simulink model "Model_6DOF_B3"  (R2020b)
settings: Solver=FixedStepAuto  StartTime=0.0  StopTime=120  FixedStep=0.05  RelTol=1e-3
values from neighbouring files (symbols this model uses):
  Ba_0 = [0 0 0 0 0 0]    [ctrl_mode_param.m]
  Bb = 4418825.3321    [load_data.m]
  Bv_0 = [tgt_speed 0 0 0 0 0]    [ctrl_mode_param.m]
  Bx_0 = [0 0 tgt_depth 0 0 0]    [ctrl_mode_param.m]
  Ixx = 5.23e7    (= 52300000)    [load_data.m]
  Ixy = 0    [load_data.m]
  Ixz = 0    [load_data.m]
  Iyy = 1.375e9    (= 1375000000)    [load_data.m]
  Iyz = 0    [load_data.m]
  Izz = 1.367e9    (= 1367000000)    [load_data.m]
  Mb = 4418825.3321    [load_data.m]
  Xb = 0    [load_data.m]
  Xg = 0    [load_data.m]
  Yb = 0    [load_data.m]
  Yg = 0    [load_data.m]
  Zb = 0.4406    [load_data.m]
  Zg = 0    [load_data.m]
undefined symbols (not defined in the file or in its folder): dA_BP1, dA_BP2, dA_Hull, dA_PH, dA_Sail, dA_SProot, dA_X1a, dA_X1b, dA_X2a, dA_X2b, dA_X3a, dA_X3b, dA_X4a, dA_X4b, its, n_BP1, n_BP2, n_Hull, n_PH, n_Sail, n_SProot, n_X1a, n_X1b, n_X2a, n_X2b, n_X3a, n_X3b, n_X4a, n_X4b, nt_BP1, nt_BP2, nt_Hull, nt_PH, nt_Sail, nt_SProot, nt_X1a, nt_X1b, nt_X2a, nt_X2b, nt_X3a, nt_X3b, nt_X4a, nt_X4b, Usp, vt1_BP1, vt1_BP2, vt1_Hull, vt1_PH, vt1_Sail, vt1_SProot, vt1_X1a, vt1_X1b, vt1_X2a, vt1_X2b, vt1_X3a, vt1_X3b, vt1_X4a, vt1_X4b, vt2_BP1, vt2_BP2 ... (+27)
libraries: simulink x5
(part 10 of 15)

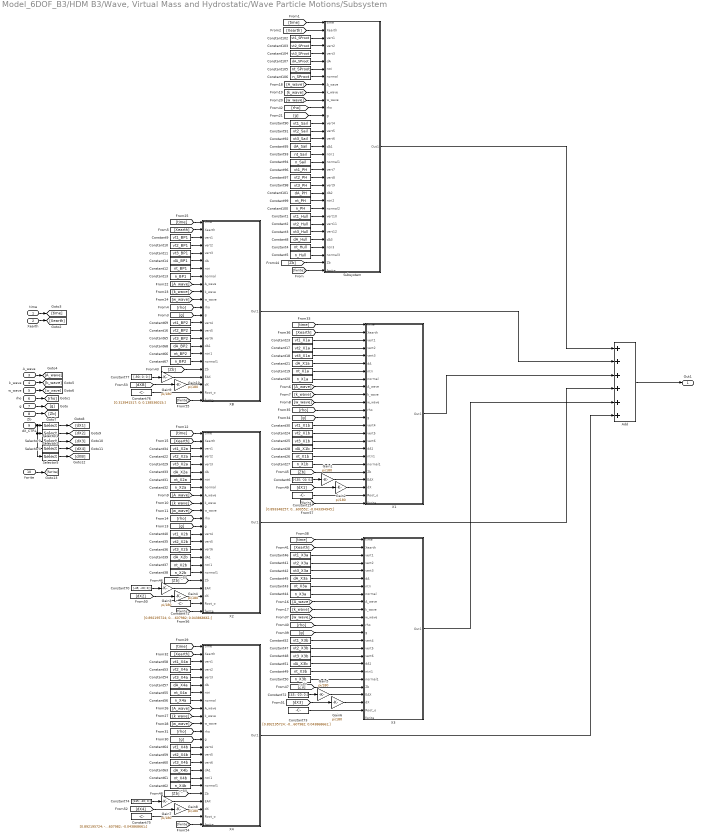
== system Model_6DOF_B3/HDM B3/Wave, Virtual Mass and Hydrostatic/Wave Particle Motions/Subsystem ==
  note: n_BP
  note: n_BP
  note: n_BP
  time : Inport
  Xearth : Inport  Port=2
  A_wave : Inport  Port=3
  k_wave : Inport  Port=4
  w_wave : Inport  Port=5
  rho : Inport  Port=6
  g : Inport  Port=7
  Zb : Inport  Port=8
  dX_CTRL : Inport  Port=9
  fwrite : Inport  Port=10
  Add : Sum  Inputs=6
  Constant1 : Constant  Value=vt1_Hull
  Constant10 : Constant  Value=vt2_BP1
  Constant100 : Constant  Value=n_PH
  Constant101 : Constant  Value=dA_PH
  Constant102 : Constant  Value=vt1_SProot
  Constant103 : Constant  Value=vt2_SProot
  Constant104 : Constant  Value=vt3_SProot
  Constant105 : Constant  Value=nt_SProot
  Constant106 : Constant  Value=n_SProot
  Constant107 : Constant  Value=dA_SProot
  Constant11 : Constant  Value=vt3_BP1
  Constant12 : Constant  Value=nt_BP1
  Constant13 : Constant  Value=n_BP1
  Constant14 : Constant  Value=dA_BP1
  Constant15 : Constant  Value=|
      | [0.893348257;
      | 0.043600552;
      | -0.043394945;]
  Constant16 : Constant  Value=vt2_BP2
  Constant17 : Constant  Value=vt2_X1a
  Constant18 : Constant  Value=vt3_X1a
  Constant19 : Constant  Value=nt_X1a
  Constant2 : Constant  Value=vt2_Hull
  Constant20 : Constant  Value=n_X1a
  Constant21 : Constant  Value=dA_X1a
  Constant22 : Constant  Value=vt2_X2a
  Constant23 : Constant  Value=vt1_X1a
  Constant24 : Constant  Value=vt2_X1b
  Constant25 : Constant  Value=vt3_X1b
  Constant26 : Constant  Value=nt_X1b
  Constant27 : Constant  Value=n_X1b
  Constant28 : Constant  Value=dA_X1b
  Constant29 : Constant  Value=vt3_X2a
  Constant3 : Constant  Value=vt3_Hull
  Constant30 : Constant  Value=vt1_X1b
  Constant31 : Constant  Value=nt_X2a
  Constant32 : Constant  Value=n_X2a
  Constant33 : Constant  Value=dA_X2a
  Constant34 : Constant  Value=vt1_X2a
  Constant35 : Constant  Value=vt2_X2b
  Constant36 : Constant  Value=vt3_X2b
  Constant37 : Constant  Value=nt_X2b
  Constant38 : Constant  Value=n_X2b
  Constant39 : Constant  Value=dA_X2b
  Constant4 : Constant  Value=nt_Hull
  Constant40 : Constant  Value=vt1_X2b
  Constant41 : Constant  Value=vt2_X3a
  Constant42 : Constant  Value=vt3_X3a
  Constant43 : Constant  Value=nt_X3a
  Constant44 : Constant  Value=n_X3a
  Constant45 : Constant  Value=dA_X3a
  Constant46 : Constant  Value=vt1_X3a
  Constant47 : Constant  Value=vt2_X3b
  Constant48 : Constant  Value=vt3_X3b
  Constant49 : Constant  Value=nt_X3b
  Constant5 : Constant  Value=n_Hull
  Constant50 : Constant  Value=n_X3b
  Constant51 : Constant  Value=dA_X3b
  Constant52 : Constant  Value=vt1_X3b
  Constant53 : Constant  Value=vt2_X4a
  Constant54 : Constant  Value=vt3_X4a
  Constant55 : Constant  Value=nt_X4a
  Constant56 : Constant  Value=n_X4a
  Constant57 : Constant  Value=dA_X4a
  Constant58 : Constant  Value=vt1_X4a
  Constant59 : Constant  Value=vt2_X4b
  Constant6 : Constant  Value=[-135; -20; 0;]
  Constant60 : Constant  Value=vt3_X4b
  Constant61 : Constant  Value=nt_X4b
  Constant62 : Constant  Value=n_X4b
  Constant63 : Constant  Value=dA_X4b
  Constant64 : Constant  Value=vt1_X4b
  Constant65 : Constant  Value=vt3_BP2
  Constant66 : Constant  Value=nt_BP2
  Constant67 : Constant  Value=n_BP2
  Constant68 : Constant  Value=dA_BP2
  Constant69 : Constant  Value=vt1_BP2
  Constant70 : Constant  Value=[-45; -20; 0;]
  Constant71 : Constant  Value=|
      | [0.892195724;
      | 0.043607982;
      | 0.043868661;]
  Constant72 : Constant  Value=[45; -20; 0;]
  Constant73 : Constant  Value=|
      | [0.892195724;
      | -0.043607982;
      | 0.043868661;]
  Constant74 : Constant  Value=[135; -20; 0;]
  Constant75 : Constant  Value=|
      | [0.892195724;
      | -0.043607982;
      | -0.043868661;]
  Constant76 : Constant  Value=|
      | [0.313941517;
      | 0;
      | 0.138536015;]
  Constant77 : Constant  Value=[-90; 0; 0;]
  Constant8 : Constant  Value=dA_Hull
  Constant9 : Constant  Value=vt1_BP1
  Constant90 : Constant  Value=vt1_Sail
  Constant91 : Constant  Value=vt2_Sail
  Constant92 : Constant  Value=vt3_Sail
  Constant93 : Constant  Value=nt_Sail
  Constant94 : Constant  Value=n_Sail
  Constant95 : Constant  Value=dA_Sail
  Constant96 : Constant  Value=vt1_PH
  Constant97 : Constant  Value=vt2_PH
  Constant98 : Constant  Value=vt3_PH
  Constant99 : Constant  Value=nt_PH
  Gain{1..10} (10 alike) : Gain  Gain=pi/180
  Selector1 : Selector  InputPortWidth=5  IndexOptions=Index vector (dialog)  Indices=1  OutputSizes=1
  Selector2 : Selector  InputPortWidth=5  IndexOptions=Index vector (dialog)  Indices=2  OutputSizes=1
  Selector3 : Selector  InputPortWidth=5  IndexOptions=Index vector (dialog)  Indices=3  OutputSizes=1
  Selector4 : Selector  InputPortWidth=5  IndexOptions=Index vector (dialog)  Indices=4  OutputSizes=1
  Selector5 : Selector  InputPortWidth=5  IndexOptions=Index vector (dialog)  Indices=5  OutputSizes=1
  Subsystem : Subsystem
  X1 : Subsystem
  X2 : Subsystem
  X3 : Subsystem
  X4 : Subsystem
  XB : Subsystem
  Out1 : Outport
  wires:
  time/1 -> [time]
  Xearth/1 -> [Xearth]
  A_wave/1 -> [A_wave]
  k_wave/1 -> [k_wave]
  w_wave/1 -> [w_wave]
  rho/1 -> [rho]
  g/1 -> [g]
  Constant94/1 -> Subsystem/19(normal1)
  Constant61/1 -> X4/18(ntri1)
  Constant57/1 -> X4/6(dA)
  [Zb] -> X4/20(Zb)
  [Zb] -> X3/20(Zb)
  Constant101/1 -> Subsystem/23(dA2)
  Constant16/1 -> XB/15(vert5)
  [Zb] -> X1/20(Zb)
  [Zb] -> X2/20(Zb)
  Constant98/1 -> Subsystem/22(vert9)
  Constant99/1 -> Subsystem/24(ntri2)
  Constant37/1 -> X2/18(ntri1)
  [Zb] -> XB/20(Zb)
  [time] -> X3/1(time)
  [Xearth] -> X1/2(Xearth)
  [w_wave] -> Subsystem/11(w_wave)
  Constant93/1 -> Subsystem/18(ntri1)
  [g] -> X2/13(g)
  Constant28/1 -> X1/17(dA1)
  [w_wave] -> X3/11(w_wave)
  Constant8/1 -> Subsystem/29(dA3)
  Constant95/1 -> Subsystem/17(dA1)
  [A_wave] -> X4/9(A_wave)
  Constant33/1 -> X2/6(dA)
  [rho] -> X4/12(rho)
  [time] -> Subsystem/1(time)
  Constant48/1 -> X3/16(vert6)
  [rho] -> Subsystem/12(rho)
  Constant60/1 -> X4/16(vert6)
  [k_wave] -> Subsystem/10(k_wave)
  Constant19/1 -> X1/7(ntri)
  [g] -> Subsystem/13(g)
  Constant102/1 -> Subsystem/3(vert1)
  Constant106/1 -> Subsystem/8(normal)
  [Xearth] -> Subsystem/2(Xearth)
  Constant107/1 -> Subsystem/6(dA)
  Constant105/1 -> Subsystem/7(ntri)
  [g] -> X4/13(g)
  Constant11/1 -> XB/5(vert3)
  Constant34/1 -> X2/3(vert1)
  Constant63/1 -> X4/17(dA1)
  [A_wave] -> X1/9(A_wave)
  Constant41/1 -> X3/4(vert2)
  [k_wave] -> X2/10(k_wave)
  Constant22/1 -> X2/4(vert2)
  Constant49/1 -> X3/18(ntri1)
  [Xearth] -> XB/2(Xearth)
  [rho] -> X2/12(rho)
  Constant27/1 -> X1/19(normal1)
  [rho] -> X3/12(rho)
  Constant55/1 -> X4/7(ntri)
  Constant45/1 -> X3/6(dA)
  Constant40/1 -> X2/14(vert4)
  Constant18/1 -> X1/5(vert3)
  [g] -> X1/13(g)
  Constant35/1 -> X2/15(vert5)
  Constant39/1 -> X2/17(dA1)
  Constant32/1 -> X2/8(normal)
  Constant47/1 -> X3/15(vert5)
  [w_wave] -> X4/11(w_wave)
  Constant44/1 -> X3/8(normal)
  [k_wave] -> X1/10(k_wave)
  Constant53/1 -> X4/4(vert2)
  [w_wave] -> XB/11(w_wave)
  [Xearth] -> X2/2(Xearth)
  [time] -> XB/1(time)
  [rho] -> XB/12(rho)
  Constant4/1 -> Subsystem/30(ntri3)
  Constant59/1 -> X4/15(vert5)
  Constant51/1 -> X3/17(dA1)
  Constant52/1 -> X3/14(vert4)
  Constant14/1 -> XB/6(dA)
  [Xearth] -> X3/2(Xearth)
  Constant25/1 -> X1/16(vert6)
  Constant67/1 -> XB/19(normal1)
  [Zb] -> Subsystem/32(Zb)
  Constant65/1 -> XB/16(vert6)
  Constant104/1 -> Subsystem/5(vert3)
  Constant13/1 -> XB/8(normal)
  Constant69/1 -> XB/14(vert4)
  Constant43/1 -> X3/7(ntri)
  [k_wave] -> X3/10(k_wave)
  [A_wave] -> X2/9(A_wave)
  Constant17/1 -> X1/4(vert2)
  [k_wave] -> XB/10(k_wave)
  Constant68/1 -> XB/17(dA1)
  Constant46/1 -> X3/3(vert1)
  Constant23/1 -> X1/3(vert1)
  Constant9/1 -> XB/3(vert1)
  Constant62/1 -> X4/19(normal1)
  [A_wave] -> XB/9(A_wave)
  Constant26/1 -> X1/18(ntri1)
  Constant56/1 -> X4/8(normal)
  Constant24/1 -> X1/15(vert5)
  Constant12/1 -> XB/7(ntri)
  Constant20/1 -> X1/8(normal)
  [g] -> X3/13(g)
  [w_wave] -> X1/11(w_wave)
  Constant100/1 -> Subsystem/25(normal2)
  Constant92/1 -> Subsystem/16(vert6)
  Constant30/1 -> X1/14(vert4)
  [time] -> X2/1(time)
  [rho] -> X1/12(rho)
  Constant91/1 -> Subsystem/15(vert5)
  [time] -> X1/1(time)
  Constant1/1 -> Subsystem/26(vert10)
  Constant31/1 -> X2/7(ntri)
  [w_wave] -> X2/11(w_wave)
  Constant21/1 -> X1/6(dA)
  Constant90/1 -> Subsystem/14(vert4)
  Constant96/1 -> Subsystem/20(vert7)
  Constant36/1 -> X2/16(vert6)
  Constant29/1 -> X2/5(vert3)
  [Xearth] -> X4/2(Xearth)
  Constant64/1 -> X4/14(vert4)
  Constant97/1 -> Subsystem/21(vert8)
  Constant2/1 -> Subsystem/27(vert11)
  Constant66/1 -> XB/18(ntri1)
  Constant54/1 -> X4/5(vert3)
  Constant38/1 -> X2/19(normal1)
  [k_wave] -> X4/10(k_wave)
  [time] -> X4/1(time)
  Constant10/1 -> XB/4(vert2)
  Constant50/1 -> X3/19(normal1)
  [A_wave] -> Subsystem/9(A_wave)
  Add/1 -> Out1/1
  Constant103/1 -> Subsystem/4(vert2)
  Constant3/1 -> Subsystem/28(vert12)
  [g] -> XB/13(g)
  Constant42/1 -> X3/5(vert3)
  Constant58/1 -> X4/3(vert1)
  Constant5/1 -> Subsystem/31(normal3)
  [A_wave] -> X3/9(A_wave)
  Zb/1 -> [Zb]
  Constant6/1 -> Gain1/1
  Gain1/1 -> X1/21(EAX)
  dX_CTRL/1 -> Selector2/1, Selector3/1, Selector5/1, Selector4/1, Selector1/1
  Selector1/1 -> [dX1]
  Selector2/1 -> [dX2]
  Selector3/1 -> [dX3]
  Selector4/1 -> [dX4]
  Selector5/1 -> [dXB]
  [dX1] -> Gain2/1
  Gain2/1 -> X1/22(dX)
  Constant15/1 -> X1/23(Root_o)
  Constant70/1 -> Gain3/1
  Gain3/1 -> X2/21(EAX)
  [dX2] -> Gain4/1
  Gain4/1 -> X2/22(dX)
  Constant71/1 -> X2/23(Root_o)
  Gain5/1 -> X3/21(EAX)
  [dX3] -> Gain6/1
  Constant72/1 -> Gain5/1
  Gain6/1 -> X3/22(dX)
  Constant73/1 -> X3/23(Root_o)
  Constant75/1 -> X4/23(Root_o)
  Gain7/1 -> X4/21(EAX)
  Constant74/1 -> Gain7/1
  [dX4] -> Gain8/1
  Gain8/1 -> X4/22(dX)
  Constant77/1 -> Gain9/1
  Gain9/1 -> XB/21(EAX)
  [dXB] -> Gain10/1
  Constant76/1 -> XB/23(Root_o)
  Gain10/1 -> XB/22(dX)
  [fwrite] -> Subsystem/33(fwrite)
  fwrite/1 -> [fwrite]
  [fwrite] -> X4/24(fwrite)
  [fwrite] -> XB/24(fwrite)
  [fwrite] -> X2/24(fwrite)
  [fwrite] -> X1/24(fwrite)
  X4/1(Out1) -> Add/6
  X3/1(Out1) -> Add/5
  X2/1(Out1) -> Add/4
  X1/1(Out1) -> Add/3
  XB/1(Out1) -> Add/2
  Subsystem/1(Out1) -> Add/1

== system Model_6DOF_B3/HDM B1/Wave, Virtual Mass and Hydrostatic/Wave Particle Motions/Subsystem/Sail Planes ==
  time : Inport
  Xearth : Inport  Port=2
  vert1 : Inport  Port=3
  vert2 : Inport  Port=4
  vert3 : Inport  Port=5
  dA : Inport  Port=6
  ntri : Inport  Port=7
  normal : Inport  Port=8
  A_wave : Inport  Port=9
  k_wave : Inport  Port=10
  w_wave : Inport  Port=11
  rho : Inport  Port=12
  g : Inport  Port=13
  vert4 : Inport  Port=14
  vert5 : Inport  Port=15
  vert6 : Inport  Port=16
  dA1 : Inport  Port=17
  ntri1 : Inport  Port=18
  normal1 : Inport  Port=19
  Zb : Inport  Port=20
  Add1 : Sum
  MATLAB Function1 : MATLAB Function  TreatAsAtomicUnit=on
  MATLAB Function2 : MATLAB Function  TreatAsAtomicUnit=on
  Mux1 : Mux  Inputs=6
  Mux2 : Mux  Inputs=6
  Out1 : Outport
  wires:
  Zb/1 -> MATLAB Function2/14(Zb), MATLAB Function1/14(Zb)
  vert6/1 -> MATLAB Function1/5(vert3)
  normal1/1 -> MATLAB Function1/8(normal)
  ntri1/1 -> MATLAB Function1/7(ntri)
  dA1/1 -> MATLAB Function1/6(dA)
  vert5/1 -> MATLAB Function1/4(vert2)
  vert2/1 -> MATLAB Function2/4(vert2)
  ntri/1 -> MATLAB Function2/7(ntri)
  normal/1 -> MATLAB Function2/8(normal)
  time/1 -> MATLAB Function2/1(time), MATLAB Function1/1(time)
  vert1/1 -> MATLAB Function2/3(vert1)
  Mux1/1 -> Add1/2
  vert3/1 -> MATLAB Function2/5(vert3)
  MATLAB Function1/6(Mz_total) -> Mux1/6
  Mux2/1 -> Add1/1
  MATLAB Function2/2(Fy_total) -> Mux2/2
  MATLAB Function2/6(Mz_total) -> Mux2/6
  g/1 -> MATLAB Function2/13(g), MATLAB Function1/13(g)
  k_wave/1 -> MATLAB Function1/10(k_wave), MATLAB Function2/10(k_wave)
  dA/1 -> MATLAB Function2/6(dA)
  vert4/1 -> MATLAB Function1/3(vert1)
  MATLAB Function2/5(My_total) -> Mux2/5
  MATLAB Function1/3(Fz_total) -> Mux1/3
  Add1/1 -> Out1/1
  MATLAB Function1/1(Fx_total) -> Mux1/1
  MATLAB Function2/1(Fx_total) -> Mux2/1
  MATLAB Function1/4(Mx_total) -> Mux1/4
  A_wave/1 -> MATLAB Function1/9(A_wave), MATLAB Function2/9(A_wave)
  rho/1 -> MATLAB Function2/12(rho), MATLAB Function1/12(rho)
  Xearth/1 -> MATLAB Function2/2(Xearth), MATLAB Function1/2(Xearth)
  MATLAB Function1/5(My_total) -> Mux1/5
  MATLAB Function1/2(Fy_total) -> Mux1/2
  w_wave/1 -> MATLAB Function2/11(w_wave), MATLAB Function1/11(w_wave)
  MATLAB Function2/4(Mx_total) -> Mux2/4
  MATLAB Function2/3(Fz_total) -> Mux2/3

== system Model_6DOF_B3/HDM B1/Wave, Virtual Mass and Hydrostatic/Wave Particle Motions/Subsystem/Subsystem ==
  time : Inport
  Xearth : Inport  Port=2
  vert1 : Inport  Port=3
  vert2 : Inport  Port=4
  vert3 : Inport  Port=5
  dA : Inport  Port=6
  ntri : Inport  Port=7
  normal : Inport  Port=8
  A_wave : Inport  Port=9
  k_wave : Inport  Port=10
  w_wave : Inport  Port=11
  rho : Inport  Port=12
  g : Inport  Port=13
  vert4 : Inport  Port=14
  vert5 : Inport  Port=15
  vert6 : Inport  Port=16
  dA1 : Inport  Port=17
  ntri1 : Inport  Port=18
  normal1 : Inport  Port=19
  vert7 : Inport  Port=20
  vert8 : Inport  Port=21
  vert9 : Inport  Port=22
  dA2 : Inport  Port=23
  ntri2 : Inport  Port=24
  normal2 : Inport  Port=25
  vert10 : Inport  Port=26
  vert11 : Inport  Port=27
  vert12 : Inport  Port=28
  dA3 : Inport  Port=29
  ntri3 : Inport  Port=30
  normal3 : Inport  Port=31
  Zb : Inport  Port=32
  Add1 : Sum  Inputs=4
  Constant : Constant
  Gain6 : Gain
  MATLAB Function1 : MATLAB Function  TreatAsAtomicUnit=on
  MATLAB Function2 : MATLAB Function  TreatAsAtomicUnit=on
  MATLAB Function3 : MATLAB Function  TreatAsAtomicUnit=on
  MATLAB Function4 : MATLAB Function  TreatAsAtomicUnit=on
  Mux{,1..3} (4 alike) : Mux  Inputs=6
  Out1 : Outport
  wires:
  Constant/1 -> MATLAB Function1/15(isample)
  Zb/1 -> MATLAB Function2/14(Zb), MATLAB Function1/14(Zb), MATLAB Function3/14(Zb), MATLAB Function4/14(Zb)
  vert8/1 -> MATLAB Function3/4(vert2)
  vert1/1 -> MATLAB Function2/3(vert1)
  vert10/1 -> MATLAB Function4/3(vert1)
  dA1/1 -> MATLAB Function1/6(dA)
  normal2/1 -> MATLAB Function3/8(normal)
  vert3/1 -> MATLAB Function2/5(vert3)
  vert6/1 -> MATLAB Function1/5(vert3)
  Add1/1 -> Out1/1
  vert2/1 -> MATLAB Function2/4(vert2)
  dA3/1 -> MATLAB Function4/6(dA)
  ntri3/1 -> MATLAB Function4/7(ntri)
  ntri2/1 -> MATLAB Function3/7(ntri)
  vert11/1 -> MATLAB Function4/4(vert2)
  MATLAB Function2/6(Mz_total) -> Mux3/6
  dA/1 -> MATLAB Function2/6(dA)
  Mux3/1 -> Gain6/1
  normal/1 -> MATLAB Function2/8(normal)
  MATLAB Function1/1(Fx_total) -> Mux1/1
  vert9/1 -> MATLAB Function3/5(vert3)
  Mux/1 -> Add1/4
  vert4/1 -> MATLAB Function1/3(vert1)
  MATLAB Function1/4(Mx_total) -> Mux1/4
  normal3/1 -> MATLAB Function4/8(normal)
  MATLAB Function3/5(My_total) -> Mux2/5
  vert12/1 -> MATLAB Function4/5(vert3)
  MATLAB Function2/1(Fx_total) -> Mux3/1
  MATLAB Function4/4(Mx_total) -> Mux/4
  dA2/1 -> MATLAB Function3/6(dA)
  MATLAB Function3/6(Mz_total) -> Mux2/6
  g/1 -> MATLAB Function2/13(g), MATLAB Function1/13(g), MATLAB Function3/13(g), MATLAB Function4/13(g)
  MATLAB Function3/3(Fz_total) -> Mux2/3
  ntri/1 -> MATLAB Function2/7(ntri)
  MATLAB Function3/2(Fy_total) -> Mux2/2
  MATLAB Function4/2(Fy_total) -> Mux/2
  Mux2/1 -> Add1/3
  MATLAB Function4/6(Mz_total) -> Mux/6
  MATLAB Function2/2(Fy_total) -> Mux3/2
  w_wave/1 -> MATLAB Function2/11(w_wave), MATLAB Function1/11(w_wave), MATLAB Function3/11(w_wave), MATLAB Function4/11(w_wave)
  MATLAB Function3/4(Mx_total) -> Mux2/4
  k_wave/1 -> MATLAB Function2/10(k_wave), MATLAB Function1/10(k_wave), MATLAB Function3/10(k_wave), MATLAB Function4/10(k_wave)
  MATLAB Function4/1(Fx_total) -> Mux/1
  MATLAB Function1/2(Fy_total) -> Mux1/2
  MATLAB Function2/3(Fz_total) -> Mux3/3
  MATLAB Function3/1(Fx_total) -> Mux2/1
  A_wave/1 -> MATLAB Function2/9(A_wave), MATLAB Function1/9(A_wave), MATLAB Function3/9(A_wave), MATLAB Function4/9(A_wave)
  MATLAB Function4/3(Fz_total) -> Mux/3
  normal1/1 -> MATLAB Function1/8(normal)
  Gain6/1 -> Add1/1
  MATLAB Function2/4(Mx_total) -> Mux3/4
  vert7/1 -> MATLAB Function3/3(vert1)
  MATLAB Function1/3(Fz_total) -> Mux1/3
  Mux1/1 -> Add1/2
  Xearth/1 -> MATLAB Function2/2(Xearth), MATLAB Function1/2(Xearth), MATLAB Function3/2(Xearth), MATLAB Function4/2(Xearth)
  MATLAB Function1/6(Mz_total) -> Mux1/6
  time/1 -> MATLAB Function2/1(time), MATLAB Function1/1(time), MATLAB Function3/1(time), MATLAB Function4/1(time)
  MATLAB Function2/5(My_total) -> Mux3/5
  MATLAB Function4/5(My_total) -> Mux/5
  vert5/1 -> MATLAB Function1/4(vert2)
  rho/1 -> MATLAB Function2/12(rho), MATLAB Function1/12(rho), MATLAB Function3/12(rho), MATLAB Function4/12(rho)
  MATLAB Function1/5(My_total) -> Mux1/5
  ntri1/1 -> MATLAB Function1/7(ntri)

== system Model_6DOF_B3/HDM B1/Wave, Virtual Mass and Hydrostatic/Wave Particle Motions/Subsystem/X1 ==
  time : Inport
  Xearth : Inport  Port=2
  vert1 : Inport  Port=3
  vert2 : Inport  Port=4
  vert3 : Inport  Port=5
  dA : Inport  Port=6
  ntri : Inport  Port=7
  normal : Inport  Port=8
  A_wave : Inport  Port=9
  k_wave : Inport  Port=10
  w_wave : Inport  Port=11
  rho : Inport  Port=12
  g : Inport  Port=13
  vert4 : Inport  Port=14
  vert5 : Inport  Port=15
  vert6 : Inport  Port=16
  dA1 : Inport  Port=17
  ntri1 : Inport  Port=18
  normal1 : Inport  Port=19
  Zb : Inport  Port=20
  Add1 : Sum
  MATLAB Function1 : MATLAB Function  TreatAsAtomicUnit=on
  MATLAB Function2 : MATLAB Function  TreatAsAtomicUnit=on
  Mux1 : Mux  Inputs=6
  Mux2 : Mux  Inputs=6
  Out1 : Outport
  wires:
  MATLAB Function1/3(Fz_total) -> Mux2/3
  MATLAB Function1/4(Mx_total) -> Mux2/4
  w_wave/1 -> MATLAB Function1/11(w_wave), MATLAB Function2/11(w_wave)
  MATLAB Function2/2(Fy_total) -> Mux1/2
  MATLAB Function2/5(My_total) -> Mux1/5
  Xearth/1 -> MATLAB Function2/2(Xearth), MATLAB Function1/2(Xearth)
  rho/1 -> MATLAB Function2/12(rho), MATLAB Function1/12(rho)
  A_wave/1 -> MATLAB Function1/9(A_wave), MATLAB Function2/9(A_wave)
  MATLAB Function2/4(Mx_total) -> Mux1/4
  MATLAB Function1/1(Fx_total) -> Mux2/1
  MATLAB Function2/1(Fx_total) -> Mux1/1
  Add1/1 -> Out1/1
  MATLAB Function2/3(Fz_total) -> Mux1/3
  MATLAB Function1/5(My_total) -> Mux2/5
  vert4/1 -> MATLAB Function2/3(vert1)
  dA/1 -> MATLAB Function1/6(dA)
  k_wave/1 -> MATLAB Function1/10(k_wave), MATLAB Function2/10(k_wave)
  g/1 -> MATLAB Function2/13(g), MATLAB Function1/13(g)
  MATLAB Function1/6(Mz_total) -> Mux2/6
  MATLAB Function1/2(Fy_total) -> Mux2/2
  Mux2/1 -> Add1/1
  MATLAB Function2/6(Mz_total) -> Mux1/6
  vert3/1 -> MATLAB Function1/5(vert3)
  Mux1/1 -> Add1/2
  vert1/1 -> MATLAB Function1/3(vert1)
  time/1 -> MATLAB Function2/1(time), MATLAB Function1/1(time)
  normal/1 -> MATLAB Function1/8(normal)
  ntri/1 -> MATLAB Function1/7(ntri)
  vert2/1 -> MATLAB Function1/4(vert2)
  vert5/1 -> MATLAB Function2/4(vert2)
  dA1/1 -> MATLAB Function2/6(dA)
  ntri1/1 -> MATLAB Function2/7(ntri)
  normal1/1 -> MATLAB Function2/8(normal)
  vert6/1 -> MATLAB Function2/5(vert3)
  Zb/1 -> MATLAB Function1/14(Zb), MATLAB Function2/14(Zb)

== system Model_6DOF_B3/HDM B1/Wave, Virtual Mass and Hydrostatic/Wave Particle Motions/Subsystem/X2 ==
  time : Inport
  Xearth : Inport  Port=2
  vert1 : Inport  Port=3
  vert2 : Inport  Port=4
  vert3 : Inport  Port=5
  dA : Inport  Port=6
  ntri : Inport  Port=7
  normal : Inport  Port=8
  A_wave : Inport  Port=9
  k_wave : Inport  Port=10
  w_wave : Inport  Port=11
  rho : Inport  Port=12
  g : Inport  Port=13
  vert4 : Inport  Port=14
  vert5 : Inport  Port=15
  vert6 : Inport  Port=16
  dA1 : Inport  Port=17
  ntri1 : Inport  Port=18
  normal1 : Inport  Port=19
  Zb : Inport  Port=20
  Add1 : Sum
  MATLAB Function1 : MATLAB Function  TreatAsAtomicUnit=on
  MATLAB Function2 : MATLAB Function  TreatAsAtomicUnit=on
  Mux1 : Mux  Inputs=6
  Mux2 : Mux  Inputs=6
  Out1 : Outport
  wires:
  Zb/1 -> MATLAB Function2/14(Zb), MATLAB Function1/14(Zb)
  vert6/1 -> MATLAB Function2/5(vert3)
  normal1/1 -> MATLAB Function2/8(normal)
  ntri1/1 -> MATLAB Function2/7(ntri)
  dA1/1 -> MATLAB Function2/6(dA)
  vert5/1 -> MATLAB Function2/4(vert2)
  vert2/1 -> MATLAB Function1/4(vert2)
  ntri/1 -> MATLAB Function1/7(ntri)
  normal/1 -> MATLAB Function1/8(normal)
  time/1 -> MATLAB Function1/1(time), MATLAB Function2/1(time)
  vert1/1 -> MATLAB Function1/3(vert1)
  Mux1/1 -> Add1/2
  vert3/1 -> MATLAB Function1/5(vert3)
  MATLAB Function2/6(Mz_total) -> Mux1/6
  Mux2/1 -> Add1/1
  MATLAB Function1/2(Fy_total) -> Mux2/2
  MATLAB Function1/6(Mz_total) -> Mux2/6
  g/1 -> MATLAB Function1/13(g), MATLAB Function2/13(g)
  k_wave/1 -> MATLAB Function2/10(k_wave), MATLAB Function1/10(k_wave)
  dA/1 -> MATLAB Function1/6(dA)
  vert4/1 -> MATLAB Function2/3(vert1)
  MATLAB Function1/5(My_total) -> Mux2/5
  MATLAB Function2/3(Fz_total) -> Mux1/3
  Add1/1 -> Out1/1
  MATLAB Function2/1(Fx_total) -> Mux1/1
  MATLAB Function1/1(Fx_total) -> Mux2/1
  MATLAB Function2/4(Mx_total) -> Mux1/4
  A_wave/1 -> MATLAB Function2/9(A_wave), MATLAB Function1/9(A_wave)
  rho/1 -> MATLAB Function1/12(rho), MATLAB Function2/12(rho)
  Xearth/1 -> MATLAB Function1/2(Xearth), MATLAB Function2/2(Xearth)
  MATLAB Function2/5(My_total) -> Mux1/5
  MATLAB Function2/2(Fy_total) -> Mux1/2
  w_wave/1 -> MATLAB Function2/11(w_wave), MATLAB Function1/11(w_wave)
  MATLAB Function1/4(Mx_total) -> Mux2/4
  MATLAB Function1/3(Fz_total) -> Mux2/3

== system Model_6DOF_B3/HDM B1/Wave, Virtual Mass and Hydrostatic/Wave Particle Motions/Subsystem/X3 ==
  time : Inport
  Xearth : Inport  Port=2
  vert1 : Inport  Port=3
  vert2 : Inport  Port=4
  vert3 : Inport  Port=5
  dA : Inport  Port=6
  ntri : Inport  Port=7
  normal : Inport  Port=8
  A_wave : Inport  Port=9
  k_wave : Inport  Port=10
  w_wave : Inport  Port=11
  rho : Inport  Port=12
  g : Inport  Port=13
  vert4 : Inport  Port=14
  vert5 : Inport  Port=15
  vert6 : Inport  Port=16
  dA1 : Inport  Port=17
  ntri1 : Inport  Port=18
  normal1 : Inport  Port=19
  Zb : Inport  Port=20
  Add1 : Sum
  MATLAB Function1 : MATLAB Function  TreatAsAtomicUnit=on
  MATLAB Function2 : MATLAB Function  TreatAsAtomicUnit=on
  Mux1 : Mux  Inputs=6
  Mux2 : Mux  Inputs=6
  Out1 : Outport
  wires:
  MATLAB Function1/3(Fz_total) -> Mux2/3
  MATLAB Function1/4(Mx_total) -> Mux2/4
  w_wave/1 -> MATLAB Function1/11(w_wave), MATLAB Function2/11(w_wave)
  MATLAB Function2/2(Fy_total) -> Mux1/2
  MATLAB Function2/5(My_total) -> Mux1/5
  Xearth/1 -> MATLAB Function2/2(Xearth), MATLAB Function1/2(Xearth)
  rho/1 -> MATLAB Function2/12(rho), MATLAB Function1/12(rho)
  A_wave/1 -> MATLAB Function1/9(A_wave), MATLAB Function2/9(A_wave)
  MATLAB Function2/4(Mx_total) -> Mux1/4
  MATLAB Function1/1(Fx_total) -> Mux2/1
  MATLAB Function2/1(Fx_total) -> Mux1/1
  Add1/1 -> Out1/1
  MATLAB Function2/3(Fz_total) -> Mux1/3
  MATLAB Function1/5(My_total) -> Mux2/5
  vert4/1 -> MATLAB Function2/3(vert1)
  dA/1 -> MATLAB Function1/6(dA)
  k_wave/1 -> MATLAB Function1/10(k_wave), MATLAB Function2/10(k_wave)
  g/1 -> MATLAB Function2/13(g), MATLAB Function1/13(g)
  MATLAB Function1/6(Mz_total) -> Mux2/6
  MATLAB Function1/2(Fy_total) -> Mux2/2
  Mux2/1 -> Add1/1
  MATLAB Function2/6(Mz_total) -> Mux1/6
  vert3/1 -> MATLAB Function1/5(vert3)
  Mux1/1 -> Add1/2
  vert1/1 -> MATLAB Function1/3(vert1)
  time/1 -> MATLAB Function2/1(time), MATLAB Function1/1(time)
  normal/1 -> MATLAB Function1/8(normal)
  ntri/1 -> MATLAB Function1/7(ntri)
  vert2/1 -> MATLAB Function1/4(vert2)
  vert5/1 -> MATLAB Function2/4(vert2)
  dA1/1 -> MATLAB Function2/6(dA)
  ntri1/1 -> MATLAB Function2/7(ntri)
  normal1/1 -> MATLAB Function2/8(normal)
  vert6/1 -> MATLAB Function2/5(vert3)
  Zb/1 -> MATLAB Function1/14(Zb), MATLAB Function2/14(Zb)

== system Model_6DOF_B3/HDM B1/Wave, Virtual Mass and Hydrostatic/Wave Particle Motions/Subsystem/X4 ==
  time : Inport
  Xearth : Inport  Port=2
  vert1 : Inport  Port=3
  vert2 : Inport  Port=4
  vert3 : Inport  Port=5
  dA : Inport  Port=6
  ntri : Inport  Port=7
  normal : Inport  Port=8
  A_wave : Inport  Port=9
  k_wave : Inport  Port=10
  w_wave : Inport  Port=11
  rho : Inport  Port=12
  g : Inport  Port=13
  vert4 : Inport  Port=14
  vert5 : Inport  Port=15
  vert6 : Inport  Port=16
  dA1 : Inport  Port=17
  ntri1 : Inport  Port=18
  normal1 : Inport  Port=19
  Zb : Inport  Port=20
  Add1 : Sum
  MATLAB Function1 : MATLAB Function  TreatAsAtomicUnit=on
  MATLAB Function2 : MATLAB Function  TreatAsAtomicUnit=on
  Mux1 : Mux  Inputs=6
  Mux2 : Mux  Inputs=6
  Out1 : Outport
  wires:
  Zb/1 -> MATLAB Function2/14(Zb), MATLAB Function1/14(Zb)
  vert6/1 -> MATLAB Function2/5(vert3)
  normal1/1 -> MATLAB Function2/8(normal)
  ntri1/1 -> MATLAB Function2/7(ntri)
  dA1/1 -> MATLAB Function2/6(dA)
  vert5/1 -> MATLAB Function2/4(vert2)
  vert2/1 -> MATLAB Function1/4(vert2)
  ntri/1 -> MATLAB Function1/7(ntri)
  normal/1 -> MATLAB Function1/8(normal)
  time/1 -> MATLAB Function1/1(time), MATLAB Function2/1(time)
  vert1/1 -> MATLAB Function1/3(vert1)
  Mux1/1 -> Add1/2
  vert3/1 -> MATLAB Function1/5(vert3)
  MATLAB Function2/6(Mz_total) -> Mux1/6
  Mux2/1 -> Add1/1
  MATLAB Function1/2(Fy_total) -> Mux2/2
  MATLAB Function1/6(Mz_total) -> Mux2/6
  g/1 -> MATLAB Function1/13(g), MATLAB Function2/13(g)
  k_wave/1 -> MATLAB Function2/10(k_wave), MATLAB Function1/10(k_wave)
  dA/1 -> MATLAB Function1/6(dA)
  vert4/1 -> MATLAB Function2/3(vert1)
  MATLAB Function1/5(My_total) -> Mux2/5
  MATLAB Function2/3(Fz_total) -> Mux1/3
  Add1/1 -> Out1/1
  MATLAB Function2/1(Fx_total) -> Mux1/1
  MATLAB Function1/1(Fx_total) -> Mux2/1
  MATLAB Function2/4(Mx_total) -> Mux1/4
  A_wave/1 -> MATLAB Function2/9(A_wave), MATLAB Function1/9(A_wave)
  rho/1 -> MATLAB Function1/12(rho), MATLAB Function2/12(rho)
  Xearth/1 -> MATLAB Function1/2(Xearth), MATLAB Function2/2(Xearth)
  MATLAB Function2/5(My_total) -> Mux1/5
  MATLAB Function2/2(Fy_total) -> Mux1/2
  w_wave/1 -> MATLAB Function2/11(w_wave), MATLAB Function1/11(w_wave)
  MATLAB Function1/4(Mx_total) -> Mux2/4
  MATLAB Function1/3(Fz_total) -> Mux2/3

== system Model_6DOF_B3/HDM B3/Wave, Virtual Mass and Hydrostatic/Wave Particle Motions/Subsystem/Subsystem ==
  time : Inport
  Xearth : Inport  Port=2
  vert1 : Inport  Port=3
  vert2 : Inport  Port=4
  vert3 : Inport  Port=5
  dA : Inport  Port=6
  ntri : Inport  Port=7
  normal : Inport  Port=8
  A_wave : Inport  Port=9
  k_wave : Inport  Port=10
  w_wave : Inport  Port=11
  rho : Inport  Port=12
  g : Inport  Port=13
  vert4 : Inport  Port=14
  vert5 : Inport  Port=15
  vert6 : Inport  Port=16
  dA1 : Inport  Port=17
  ntri1 : Inport  Port=18
  normal1 : Inport  Port=19
  vert7 : Inport  Port=20
  vert8 : Inport  Port=21
  vert9 : Inport  Port=22
  dA2 : Inport  Port=23
  ntri2 : Inport  Port=24
  normal2 : Inport  Port=25
  vert10 : Inport  Port=26
  vert11 : Inport  Port=27
  vert12 : Inport  Port=28
  dA3 : Inport  Port=29
  ntri3 : Inport  Port=30
  normal3 : Inport  Port=31
  Zb : Inport  Port=32
  fwrite : Inport  Port=33
  Add1 : Sum  Inputs=4
  Constant{1..4} (4 alike) : Constant  Value=its
  Gain6 : Gain
  MATLAB Function1 : MATLAB Function  TreatAsAtomicUnit=on
  MATLAB Function3 : MATLAB Function  TreatAsAtomicUnit=on
  MATLAB Function4 : MATLAB Function  TreatAsAtomicUnit=on
  MATLAB Function5 : MATLAB Function  TreatAsAtomicUnit=on
  Mux{1..4} (4 alike) : Mux  Inputs=6
  Out1 : Outport
  wires:
  ntri1/1 -> MATLAB Function1/7(ntri)
  rho/1 -> MATLAB Function5/12(rho), MATLAB Function1/12(rho), MATLAB Function4/12(rho), MATLAB Function3/12(rho)
  vert5/1 -> MATLAB Function1/4(vert2)
  MATLAB Function5/5(My_total) -> Mux3/5
  time/1 -> MATLAB Function5/1(time), MATLAB Function1/1(time), MATLAB Function4/1(time), MATLAB Function3/1(time)
  Xearth/1 -> MATLAB Function5/2(Xearth), MATLAB Function1/2(Xearth), MATLAB Function4/2(Xearth), MATLAB Function3/2(Xearth)
  vert7/1 -> MATLAB Function3/3(vert1)
  MATLAB Function5/4(Mx_total) -> Mux3/4
  Gain6/1 -> Add1/1
  normal1/1 -> MATLAB Function1/8(normal)
  A_wave/1 -> MATLAB Function5/9(A_wave), MATLAB Function1/9(A_wave), MATLAB Function4/9(A_wave), MATLAB Function3/9(A_wave)
  MATLAB Function5/3(Fz_total) -> Mux3/3
  k_wave/1 -> MATLAB Function5/10(k_wave), MATLAB Function1/10(k_wave), MATLAB Function4/10(k_wave), MATLAB Function3/10(k_wave)
  w_wave/1 -> MATLAB Function5/11(w_wave), MATLAB Function1/11(w_wave), MATLAB Function4/11(w_wave), MATLAB Function3/11(w_wave)
  MATLAB Function5/2(Fy_total) -> Mux3/2
  ntri/1 -> MATLAB Function5/7(ntri)
  g/1 -> MATLAB Function5/13(g), MATLAB Function1/13(g), MATLAB Function4/13(g), MATLAB Function3/13(g)
  dA2/1 -> MATLAB Function3/6(dA)
  MATLAB Function5/1(Fx_total) -> Mux3/1
  vert12/1 -> MATLAB Function4/5(vert3)
  normal3/1 -> MATLAB Function4/8(normal)
  vert4/1 -> MATLAB Function1/3(vert1)
  vert9/1 -> MATLAB Function3/5(vert3)
  normal/1 -> MATLAB Function5/8(normal)
  Mux3/1 -> Gain6/1
  dA/1 -> MATLAB Function5/6(dA)
  MATLAB Function5/6(Mz_total) -> Mux3/6
  vert11/1 -> MATLAB Function4/4(vert2)
  ntri2/1 -> MATLAB Function3/7(ntri)
  ntri3/1 -> MATLAB Function4/7(ntri)
  dA3/1 -> MATLAB Function4/6(dA)
  vert2/1 -> MATLAB Function5/4(vert2)
  Add1/1 -> Out1/1
  vert6/1 -> MATLAB Function1/5(vert3)
  vert3/1 -> MATLAB Function5/5(vert3)
  normal2/1 -> MATLAB Function3/8(normal)
  dA1/1 -> MATLAB Function1/6(dA)
  vert10/1 -> MATLAB Function4/3(vert1)
  vert1/1 -> MATLAB Function5/3(vert1)
  vert8/1 -> MATLAB Function3/4(vert2)
  Zb/1 -> MATLAB Function5/14(Zb), MATLAB Function1/14(Zb), MATLAB Function3/14(Zb), MATLAB Function4/14(Zb)
  Constant2/1 -> MATLAB Function1/15(its)
  Constant1/1 -> MATLAB Function5/15(its)
  Constant3/1 -> MATLAB Function3/15(its)
  Constant4/1 -> MATLAB Function4/15(its)
  fwrite/1 -> MATLAB Function5/16(fwrite), MATLAB Function1/16(fwrite), MATLAB Function4/16(fwrite), MATLAB Function3/16(fwrite)
  Mux2/1 -> Add1/3
  MATLAB Function1/6(Mz_total) -> Mux1/6
  Mux1/1 -> Add1/2
  MATLAB Function1/1(Fx_total) -> Mux1/1
  MATLAB Function1/2(Fy_total) -> Mux1/2
  MATLAB Function1/3(Fz_total) -> Mux1/3
  MATLAB Function1/4(Mx_total) -> Mux1/4
  MATLAB Function1/5(My_total) -> Mux1/5
  MATLAB Function3/5(My_total) -> Mux2/5
  MATLAB Function3/4(Mx_total) -> Mux2/4
  MATLAB Function3/3(Fz_total) -> Mux2/3
  MATLAB Function3/2(Fy_total) -> Mux2/2
  MATLAB Function3/1(Fx_total) -> Mux2/1
  MATLAB Function3/6(Mz_total) -> Mux2/6
  MATLAB Function4/6(Mz_total) -> Mux4/6
  MATLAB Function4/1(Fx_total) -> Mux4/1
  MATLAB Function4/2(Fy_total) -> Mux4/2
  MATLAB Function4/3(Fz_total) -> Mux4/3
  MATLAB Function4/4(Mx_total) -> Mux4/4
  MATLAB Function4/5(My_total) -> Mux4/5
  Mux4/1 -> Add1/4

== system Model_6DOF_B3/HDM B3/Wave, Virtual Mass and Hydrostatic/Wave Particle Motions/Subsystem/X1 ==
  time : Inport
  Xearth : Inport  Port=2
  vert1 : Inport  Port=3
  vert2 : Inport  Port=4
  vert3 : Inport  Port=5
  dA : Inport  Port=6
  ntri : Inport  Port=7
  normal : Inport  Port=8
  A_wave : Inport  Port=9
  k_wave : Inport  Port=10
  w_wave : Inport  Port=11
  rho : Inport  Port=12
  g : Inport  Port=13
  vert4 : Inport  Port=14
  vert5 : Inport  Port=15
  vert6 : Inport  Port=16
  dA1 : Inport  Port=17
  ntri1 : Inport  Port=18
  normal1 : Inport  Port=19
  Zb : Inport  Port=20
  EAX : Inport  Port=21
  dX : Inport  Port=22
  Root_o : Inport  Port=23
  fwrite : Inport  Port=24
  Add1 : Sum
  CG : Constant  Value=[32.3114; 0; 0;]
  Constant : Constant  Value=its
  MATLAB Function1 : MATLAB Function  TreatAsAtomicUnit=on
  MATLAB Function4 : MATLAB Function  TreatAsAtomicUnit=on
  Mux1 : Mux  Inputs=6
  Mux2 : Mux  Inputs=6
  Out1 : Outport
  wires:
  Zb/1 -> MATLAB Function1/14(Zb), MATLAB Function4/14(Zb)
  vert2/1 -> MATLAB Function4/4(vert2)
  ntri/1 -> MATLAB Function4/7(ntri)
  normal/1 -> MATLAB Function4/8(normal)
  time/1 -> MATLAB Function1/1(time), MATLAB Function4/1(time)
  vert1/1 -> MATLAB Function4/3(vert1)
  Mux1/1 -> Add1/2
  vert3/1 -> MATLAB Function4/5(vert3)
  Mux2/1 -> Add1/1
  MATLAB Function4/2(Fy_total) -> Mux2/2
  MATLAB Function4/6(Mz_total) -> Mux2/6
  g/1 -> MATLAB Function4/13(g), MATLAB Function1/13(g)
  k_wave/1 -> MATLAB Function4/10(k_wave), MATLAB Function1/10(k_wave)
  dA/1 -> MATLAB Function4/6(dA)
  MATLAB Function4/5(My_total) -> Mux2/5
  MATLAB Function1/3(Fz_total) -> Mux1/3
  Add1/1 -> Out1/1
  MATLAB Function1/1(Fx_total) -> Mux1/1
  MATLAB Function4/1(Fx_total) -> Mux2/1
  MATLAB Function1/4(Mx_total) -> Mux1/4
  A_wave/1 -> MATLAB Function4/9(A_wave), MATLAB Function1/9(A_wave)
  rho/1 -> MATLAB Function4/12(rho), MATLAB Function1/12(rho)
  Xearth/1 -> MATLAB Function4/2(Xearth), MATLAB Function1/2(Xearth)
  MATLAB Function1/2(Fy_total) -> Mux1/2
  w_wave/1 -> MATLAB Function4/11(w_wave), MATLAB Function1/11(w_wave)
  MATLAB Function4/4(Mx_total) -> Mux2/4
  MATLAB Function4/3(Fz_total) -> Mux2/3
  EAX/1 -> MATLAB Function1/15(EAX), MATLAB Function4/15(EAX)
  dX/1 -> MATLAB Function1/16(dX), MATLAB Function4/16(dX)
  Constant/1 -> MATLAB Function4/17(its), MATLAB Function1/17(its)
  Root_o/1 -> MATLAB Function4/18(origin), MATLAB Function1/18(origin)
  CG/1 -> MATLAB Function1/19(xcg), MATLAB Function4/19(xcg)
  MATLAB Function1/5(My_total) -> Mux1/5
  MATLAB Function1/6(Mz_total) -> Mux1/6
  vert4/1 -> MATLAB Function1/3(vert1)
  vert5/1 -> MATLAB Function1/4(vert2)
  vert6/1 -> MATLAB Function1/5(vert3)
  dA1/1 -> MATLAB Function1/6(dA)
  ntri1/1 -> MATLAB Function1/7(ntri)
  normal1/1 -> MATLAB Function1/8(normal)
  fwrite/1 -> MATLAB Function1/20(fwrite), MATLAB Function4/20(fwrite)

== system Model_6DOF_B3/HDM B3/Wave, Virtual Mass and Hydrostatic/Wave Particle Motions/Subsystem/X2 ==
  time : Inport
  Xearth : Inport  Port=2
  vert1 : Inport  Port=3
  vert2 : Inport  Port=4
  vert3 : Inport  Port=5
  dA : Inport  Port=6
  ntri : Inport  Port=7
  normal : Inport  Port=8
  A_wave : Inport  Port=9
  k_wave : Inport  Port=10
  w_wave : Inport  Port=11
  rho : Inport  Port=12
  g : Inport  Port=13
  vert4 : Inport  Port=14
  vert5 : Inport  Port=15
  vert6 : Inport  Port=16
  dA1 : Inport  Port=17
  ntri1 : Inport  Port=18
  normal1 : Inport  Port=19
  Zb : Inport  Port=20
  EAX : Inport  Port=21
  dX : Inport  Port=22
  Root_o : Inport  Port=23
  fwrite : Inport  Port=24
  Add1 : Sum
  CG : Constant  Value=[32.3114; 0; 0;]
  Constant : Constant  Value=its
  MATLAB Function1 : MATLAB Function  TreatAsAtomicUnit=on
  MATLAB Function4 : MATLAB Function  TreatAsAtomicUnit=on
  Mux1 : Mux  Inputs=6
  Mux2 : Mux  Inputs=6
  Out1 : Outport
  wires:
  Zb/1 -> MATLAB Function4/14(Zb), MATLAB Function1/14(Zb)
  vert2/1 -> MATLAB Function4/4(vert2)
  ntri/1 -> MATLAB Function4/7(ntri)
  normal/1 -> MATLAB Function4/8(normal)
  time/1 -> MATLAB Function1/1(time), MATLAB Function4/1(time)
  vert1/1 -> MATLAB Function4/3(vert1)
  Mux1/1 -> Add1/2
  vert3/1 -> MATLAB Function4/5(vert3)
  Mux2/1 -> Add1/1
  MATLAB Function4/2(Fy_total) -> Mux2/2
  MATLAB Function4/6(Mz_total) -> Mux2/6
  g/1 -> MATLAB Function4/13(g), MATLAB Function1/13(g)
  k_wave/1 -> MATLAB Function4/10(k_wave), MATLAB Function1/10(k_wave)
  dA/1 -> MATLAB Function4/6(dA)
  MATLAB Function4/5(My_total) -> Mux2/5
  MATLAB Function1/3(Fz_total) -> Mux1/3
  Add1/1 -> Out1/1
  MATLAB Function1/1(Fx_total) -> Mux1/1
  MATLAB Function4/1(Fx_total) -> Mux2/1
  MATLAB Function1/4(Mx_total) -> Mux1/4
  A_wave/1 -> MATLAB Function4/9(A_wave), MATLAB Function1/9(A_wave)
  rho/1 -> MATLAB Function4/12(rho), MATLAB Function1/12(rho)
  Xearth/1 -> MATLAB Function4/2(Xearth), MATLAB Function1/2(Xearth)
  MATLAB Function1/2(Fy_total) -> Mux1/2
  w_wave/1 -> MATLAB Function4/11(w_wave), MATLAB Function1/11(w_wave)
  MATLAB Function4/4(Mx_total) -> Mux2/4
  MATLAB Function4/3(Fz_total) -> Mux2/3
  EAX/1 -> MATLAB Function4/15(EAX), MATLAB Function1/15(EAX)
  dX/1 -> MATLAB Function4/16(dX), MATLAB Function1/16(dX)
  Constant/1 -> MATLAB Function4/17(its), MATLAB Function1/17(its)
  Root_o/1 -> MATLAB Function1/18(origin), MATLAB Function4/18(origin)
  CG/1 -> MATLAB Function4/19(xcg), MATLAB Function1/19(xcg)
  MATLAB Function1/5(My_total) -> Mux1/5
  MATLAB Function1/6(Mz_total) -> Mux1/6
  fwrite/1 -> MATLAB Function4/20(fwrite), MATLAB Function1/20(fwrite)
  vert4/1 -> MATLAB Function1/3(vert1)
  vert5/1 -> MATLAB Function1/4(vert2)
  vert6/1 -> MATLAB Function1/5(vert3)
  dA1/1 -> MATLAB Function1/6(dA)
  ntri1/1 -> MATLAB Function1/7(ntri)
  normal1/1 -> MATLAB Function1/8(normal)

== system Model_6DOF_B3/HDM B3/Wave, Virtual Mass and Hydrostatic/Wave Particle Motions/Subsystem/X3 ==
  time : Inport
  Xearth : Inport  Port=2
  vert1 : Inport  Port=3
  vert2 : Inport  Port=4
  vert3 : Inport  Port=5
  dA : Inport  Port=6
  ntri : Inport  Port=7
  normal : Inport  Port=8
  A_wave : Inport  Port=9
  k_wave : Inport  Port=10
  w_wave : Inport  Port=11
  rho : Inport  Port=12
  g : Inport  Port=13
  vert4 : Inport  Port=14
  vert5 : Inport  Port=15
  vert6 : Inport  Port=16
  dA1 : Inport  Port=17
  ntri1 : Inport  Port=18
  normal1 : Inport  Port=19
  Zb : Inport  Port=20
  EAX : Inport  Port=21
  dX : Inport  Port=22
  Root_o : Inport  Port=23
  fwrite : Inport  Port=24
  Add1 : Sum
  CG : Constant  Value=[32.3114; 0; 0;]
  Constant : Constant  Value=its
  MATLAB Function1 : MATLAB Function  TreatAsAtomicUnit=on
  MATLAB Function4 : MATLAB Function  TreatAsAtomicUnit=on
  Mux1 : Mux  Inputs=6
  Mux2 : Mux  Inputs=6
  Out1 : Outport
  wires:
  MATLAB Function1/6(Mz_total) -> Mux1/6
  MATLAB Function1/5(My_total) -> Mux1/5
  CG/1 -> MATLAB Function1/19(xcg), MATLAB Function4/19(xcg)
  Root_o/1 -> MATLAB Function1/18(origin), MATLAB Function4/18(origin)
  Constant/1 -> MATLAB Function1/17(its), MATLAB Function4/17(its)
  dX/1 -> MATLAB Function1/16(dX), MATLAB Function4/16(dX)
  EAX/1 -> MATLAB Function1/15(EAX), MATLAB Function4/15(EAX)
  MATLAB Function4/3(Fz_total) -> Mux2/3
  MATLAB Function4/4(Mx_total) -> Mux2/4
  w_wave/1 -> MATLAB Function4/11(w_wave), MATLAB Function1/11(w_wave)
  MATLAB Function1/2(Fy_total) -> Mux1/2
  Xearth/1 -> MATLAB Function4/2(Xearth), MATLAB Function1/2(Xearth)
  rho/1 -> MATLAB Function4/12(rho), MATLAB Function1/12(rho)
  A_wave/1 -> MATLAB Function4/9(A_wave), MATLAB Function1/9(A_wave)
  MATLAB Function1/4(Mx_total) -> Mux1/4
  MATLAB Function4/1(Fx_total) -> Mux2/1
  MATLAB Function1/1(Fx_total) -> Mux1/1
  Add1/1 -> Out1/1
  MATLAB Function1/3(Fz_total) -> Mux1/3
  MATLAB Function4/5(My_total) -> Mux2/5
  dA/1 -> MATLAB Function4/6(dA)
  k_wave/1 -> MATLAB Function4/10(k_wave), MATLAB Function1/10(k_wave)
  g/1 -> MATLAB Function1/13(g), MATLAB Function4/13(g)
  MATLAB Function4/6(Mz_total) -> Mux2/6
  MATLAB Function4/2(Fy_total) -> Mux2/2
  Mux2/1 -> Add1/1
  vert3/1 -> MATLAB Function4/5(vert3)
  Mux1/1 -> Add1/2
  vert1/1 -> MATLAB Function4/3(vert1)
  time/1 -> MATLAB Function1/1(time), MATLAB Function4/1(time)
  normal/1 -> MATLAB Function4/8(normal)
  ntri/1 -> MATLAB Function4/7(ntri)
  vert2/1 -> MATLAB Function4/4(vert2)
  Zb/1 -> MATLAB Function4/14(Zb), MATLAB Function1/14(Zb)
  vert4/1 -> MATLAB Function1/3(vert1)
  vert5/1 -> MATLAB Function1/4(vert2)
  vert6/1 -> MATLAB Function1/5(vert3)
  dA1/1 -> MATLAB Function1/6(dA)
  ntri1/1 -> MATLAB Function1/7(ntri)
  normal1/1 -> MATLAB Function1/8(normal)
  fwrite/1 -> MATLAB Function1/20(fwrite), MATLAB Function4/20(fwrite)

== system Model_6DOF_B3/HDM B3/Wave, Virtual Mass and Hydrostatic/Wave Particle Motions/Subsystem/X4 ==
  time : Inport
  Xearth : Inport  Port=2
  vert1 : Inport  Port=3
  vert2 : Inport  Port=4
  vert3 : Inport  Port=5
  dA : Inport  Port=6
  ntri : Inport  Port=7
  normal : Inport  Port=8
  A_wave : Inport  Port=9
  k_wave : Inport  Port=10
  w_wave : Inport  Port=11
  rho : Inport  Port=12
  g : Inport  Port=13
  vert4 : Inport  Port=14
  vert5 : Inport  Port=15
  vert6 : Inport  Port=16
  dA1 : Inport  Port=17
  ntri1 : Inport  Port=18
  normal1 : Inport  Port=19
  Zb : Inport  Port=20
  EAX : Inport  Port=21
  dX : Inport  Port=22
  Root_o : Inport  Port=23
  fwrite : Inport  Port=24
  Add1 : Sum
  CG : Constant  Value=[32.3114; 0; 0;]
  Constant : Constant  Value=its
  MATLAB Function1 : MATLAB Function  TreatAsAtomicUnit=on
  MATLAB Function4 : MATLAB Function  TreatAsAtomicUnit=on
  Mux1 : Mux  Inputs=6
  Mux2 : Mux  Inputs=6
  Out1 : Outport
  wires:
  Zb/1 -> MATLAB Function1/14(Zb), MATLAB Function4/14(Zb)
  vert6/1 -> MATLAB Function1/5(vert3)
  normal1/1 -> MATLAB Function1/8(normal)
  ntri1/1 -> MATLAB Function1/7(ntri)
  dA1/1 -> MATLAB Function1/6(dA)
  vert5/1 -> MATLAB Function1/4(vert2)
  vert2/1 -> MATLAB Function4/4(vert2)
  ntri/1 -> MATLAB Function4/7(ntri)
  normal/1 -> MATLAB Function4/8(normal)
  time/1 -> MATLAB Function1/1(time), MATLAB Function4/1(time)
  vert1/1 -> MATLAB Function4/3(vert1)
  Mux1/1 -> Add1/2
  vert3/1 -> MATLAB Function4/5(vert3)
  Mux2/1 -> Add1/1
  MATLAB Function4/2(Fy_total) -> Mux2/2
  MATLAB Function4/6(Mz_total) -> Mux2/6
  g/1 -> MATLAB Function4/13(g), MATLAB Function1/13(g)
  k_wave/1 -> MATLAB Function4/10(k_wave), MATLAB Function1/10(k_wave)
  dA/1 -> MATLAB Function4/6(dA)
  vert4/1 -> MATLAB Function1/3(vert1)
  MATLAB Function4/5(My_total) -> Mux2/5
  MATLAB Function1/3(Fz_total) -> Mux1/3
  Add1/1 -> Out1/1
  MATLAB Function1/1(Fx_total) -> Mux1/1
  MATLAB Function4/1(Fx_total) -> Mux2/1
  MATLAB Function1/4(Mx_total) -> Mux1/4
  A_wave/1 -> MATLAB Function4/9(A_wave), MATLAB Function1/9(A_wave)
  rho/1 -> MATLAB Function4/12(rho), MATLAB Function1/12(rho)
  Xearth/1 -> MATLAB Function1/2(Xearth), MATLAB Function4/2(Xearth)
  MATLAB Function1/2(Fy_total) -> Mux1/2
  w_wave/1 -> MATLAB Function4/11(w_wave), MATLAB Function1/11(w_wave)
  MATLAB Function4/4(Mx_total) -> Mux2/4
  MATLAB Function4/3(Fz_total) -> Mux2/3
  EAX/1 -> MATLAB Function1/15(EAX), MATLAB Function4/15(EAX)
  dX/1 -> MATLAB Function1/16(dX), MATLAB Function4/16(dX)
  Constant/1 -> MATLAB Function1/17(its), MATLAB Function4/17(its)
  Root_o/1 -> MATLAB Function1/18(origin), MATLAB Function4/18(origin)
  CG/1 -> MATLAB Function1/19(xcg), MATLAB Function4/19(xcg)
  MATLAB Function1/5(My_total) -> Mux1/5
  MATLAB Function1/6(Mz_total) -> Mux1/6
  fwrite/1 -> MATLAB Function1/20(fwrite), MATLAB Function4/20(fwrite)

== system Model_6DOF_B3/HDM B3/Wave, Virtual Mass and Hydrostatic/Wave Particle Motions/Subsystem/XB ==
  time : Inport
  Xearth : Inport  Port=2
  vert1 : Inport  Port=3
  vert2 : Inport  Port=4
  vert3 : Inport  Port=5
  dA : Inport  Port=6
  ntri : Inport  Port=7
  normal : Inport  Port=8
  A_wave : Inport  Port=9
  k_wave : Inport  Port=10
  w_wave : Inport  Port=11
  rho : Inport  Port=12
  g : Inport  Port=13
  vert4 : Inport  Port=14
  vert5 : Inport  Port=15
  vert6 : Inport  Port=16
  dA1 : Inport  Port=17
  ntri1 : Inport  Port=18
  normal1 : Inport  Port=19
  Zb : Inport  Port=20
  EAX : Inport  Port=21
  dX : Inport  Port=22
  Root_o : Inport  Port=23
  fwrite : Inport  Port=24
  Add1 : Sum
  CG : Constant  Value=[32.3114; 0; 0;]
  Constant : Constant  Value=its
  MATLAB Function1 : MATLAB Function  TreatAsAtomicUnit=on
  MATLAB Function4 : MATLAB Function  TreatAsAtomicUnit=on
  Mux1 : Mux  Inputs=6
  Mux2 : Mux  Inputs=6
  Out1 : Outport
  wires:
  MATLAB Function1/6(Mz_total) -> Mux1/6
  MATLAB Function1/5(My_total) -> Mux1/5
  CG/1 -> MATLAB Function4/19(xcg), MATLAB Function1/19(xcg)
  Root_o/1 -> MATLAB Function4/18(origin), MATLAB Function1/18(origin)
  Constant/1 -> MATLAB Function4/17(its), MATLAB Function1/17(its)
  dX/1 -> MATLAB Function4/16(dX), MATLAB Function1/16(dX)
  EAX/1 -> MATLAB Function4/15(EAX), MATLAB Function1/15(EAX)
  MATLAB Function4/3(Fz_total) -> Mux2/3
  MATLAB Function4/4(Mx_total) -> Mux2/4
  w_wave/1 -> MATLAB Function4/11(w_wave), MATLAB Function1/11(w_wave)
  MATLAB Function1/2(Fy_total) -> Mux1/2
  Xearth/1 -> MATLAB Function4/2(Xearth), MATLAB Function1/2(Xearth)
  rho/1 -> MATLAB Function4/12(rho), MATLAB Function1/12(rho)
  A_wave/1 -> MATLAB Function4/9(A_wave), MATLAB Function1/9(A_wave)
  MATLAB Function1/4(Mx_total) -> Mux1/4
  MATLAB Function4/1(Fx_total) -> Mux2/1
  MATLAB Function1/1(Fx_total) -> Mux1/1
  Add1/1 -> Out1/1
  MATLAB Function1/3(Fz_total) -> Mux1/3
  MATLAB Function4/5(My_total) -> Mux2/5
  dA/1 -> MATLAB Function4/6(dA)
  k_wave/1 -> MATLAB Function4/10(k_wave), MATLAB Function1/10(k_wave)
  g/1 -> MATLAB Function4/13(g), MATLAB Function1/13(g)
  MATLAB Function4/6(Mz_total) -> Mux2/6
  MATLAB Function4/2(Fy_total) -> Mux2/2
  Mux2/1 -> Add1/1
  vert3/1 -> MATLAB Function4/5(vert3)
  Mux1/1 -> Add1/2
  vert1/1 -> MATLAB Function4/3(vert1)
  time/1 -> MATLAB Function1/1(time), MATLAB Function4/1(time)
  normal/1 -> MATLAB Function4/8(normal)
  ntri/1 -> MATLAB Function4/7(ntri)
  vert2/1 -> MATLAB Function4/4(vert2)
  Zb/1 -> MATLAB Function4/14(Zb), MATLAB Function1/14(Zb)
  vert4/1 -> MATLAB Function1/3(vert1)
  vert5/1 -> MATLAB Function1/4(vert2)
  vert6/1 -> MATLAB Function1/5(vert3)
  dA1/1 -> MATLAB Function1/6(dA)
  ntri1/1 -> MATLAB Function1/7(ntri)
  normal1/1 -> MATLAB Function1/8(normal)
  fwrite/1 -> MATLAB Function4/20(fwrite), MATLAB Function1/20(fwrite)
